simulink model "FSFB_FF_Sim"  (R2022a)
settings: Solver=VariableStepAuto  StartTime=tspan(1)  StopTime=tspan(2)  RelTol=1e-7
undefined symbols (not defined in the file): r_sim
settings Model: Creator=domin  LastModifiedBy=domin
settings SolverCC: AlgebraicLoopSolver=TrustRegion
settings DebuggingCC: AlgebraicLoopMsg=none  UnconnectedInputMsg=warning  UnconnectedOutputMsg=warning  UnconnectedLineMsg=warning  ModelReferenceExtraNoncontSigs=none  SFMachineParentedDataDiag=warning
settings RTWCC: DLArmComputeVersion=19.05

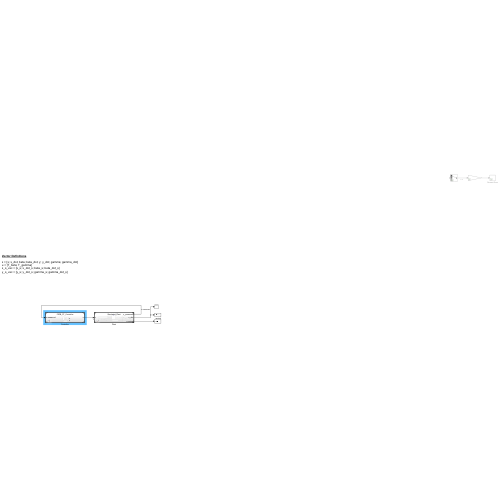
[thumbnail: Simulink's stored preview of the top-level diagram]
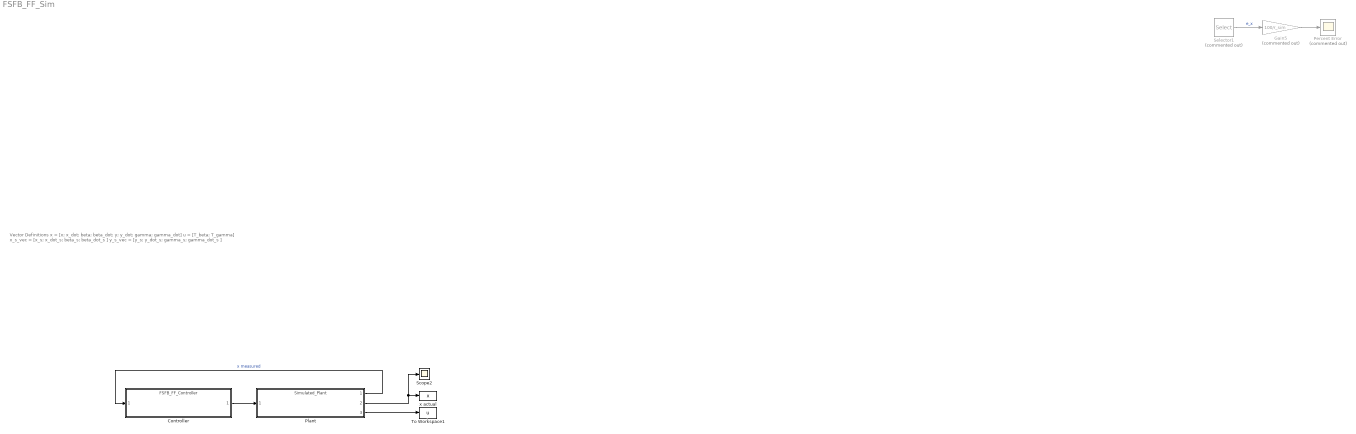
== system FSFB_FF_Sim ==
  note: Vector Definitions
      |
      | x = [x; x_dot; beta; beta_dot; y; y_dot; gamma; gamma_dot]
      | u = [T_beta; T_gamma]
      | x_s_vec = [x_s; x_dot_s; beta_s; beta_dot_s ]
      | y_s_vec = [y_s; y_dot_s; gamma_s; gamma_dot_s ]
  Controller : ModelReference  ModelNameDialog=FSFB_FF_Controller.slx  SimulationMode=Normal  ModelReferenceVersion=1.86
  Gain5 : Gain  Commented=on  Gain=100/r_sim
  Percent Error : Scope  Commented=on
  Plant : ModelReference  ModelNameDialog=Simulated_Plant.slx  SimulationMode=Normal  ModelReferenceVersion=2.30
  Scope2 : Scope
  Selector1 : Selector  Commented=on  InputPortWidth=5  IndexOptions=Index vector (dialog)  Indices=[1]  OutputSizes=1
  To Workspace1 : ToWorkspace  VariableName=u  SampleTime=-1
  x actual : ToWorkspace  VariableName=x  SampleTime=-1
  wires:
  Gain5/1 -> Percent Error/1
  Selector1/1 -> Gain5/1  "e_x"
  Plant/3 -> To Workspace1/1
  Plant/2 -> Scope2/1, x actual/1
  Controller/1 -> Plant/1
  Plant/1 -> Controller/1  "x measured"
